simulink library "pixhawk_slib_rfly"  (R2022b)
settings: Solver=ode45  StartTime=0.0  StopTime=10.0  RelTol=1e-3
libraries: pixhawk_slib_uORB_RW x44, $bdroot x7
(part 1 of 2)
settings Model: Creator=skuznick  LastModifiedBy=uavcs
settings SolverCC: AlgebraicLoopSolver=TrustRegion
settings DataIOCC: LimitDataPoints=on  SaveFormat=Array  ReturnWorkspaceOutputs=off
settings OptimizationCC: BlockReduction=off  BooleanDataType=off  LifeSpan=inf
settings DebuggingCC: SaveWithParameterizedLinksMsg=none  UnderspecifiedInitializationDetection=Classic  MergeDetectMultiDrivingBlocksExec=none  SignalResolutionControl=TryResolveAllWithWarning  UnconnectedInputMsg=warning  UnconnectedOutputMsg=warning  UnconnectedLineMsg=warning  AllowSymbolicDim=off  SFUnexpectedBacktrackingDiag=warning  SFNoUnconditionalDefaultTransitionDiag=warning  SFExecutionAtInitializationDiag=none  SFMachineParentedDataDiag=warning  ArithmeticOperatorsInVariantConditions=warning
settings HardwareCC: ProdBitPerPointer=32  ProdBitPerSizeT=32  ProdBitPerPtrDiffT=32  ProdLargestAtomicFloat=None  ProdIntDivRoundTo=Undefined  ProdEndianess=Unspecified  ProdWordSize=32  ProdHWDeviceType=32-bit Generic  TargetUnknown=on
settings ModelReferenceCC: EnableRefExpFcnMdlSchedulingChecks=on  PropagateSignalLabelsOutOfModel=off
settings SFSimCC: SimUseLocalCustomCode=off  CustomCodeUndefinedFunction=UseInterfaceOnly
settings RTWCC: RTWUseLocalCustomCode=off
settings CodeAppCC: StateflowObjectComments=on
settings GRTTargetCC: TargetLangStandard=C89/C90 (ANSI)
settings ConfigComp: CovMetricSettings=dw  CovSaveCumulativeToWorkspaceVar=on  CovSaveSingleToWorkspaceVar=on  CovExternalEMLEnable=off  CovSFcnEnable=off

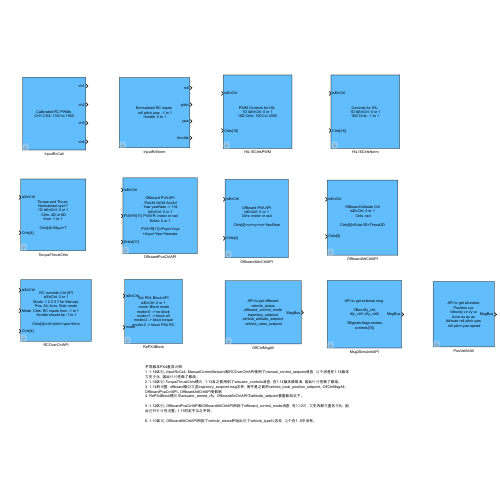
[thumbnail: Simulink's stored preview of the top-level diagram]
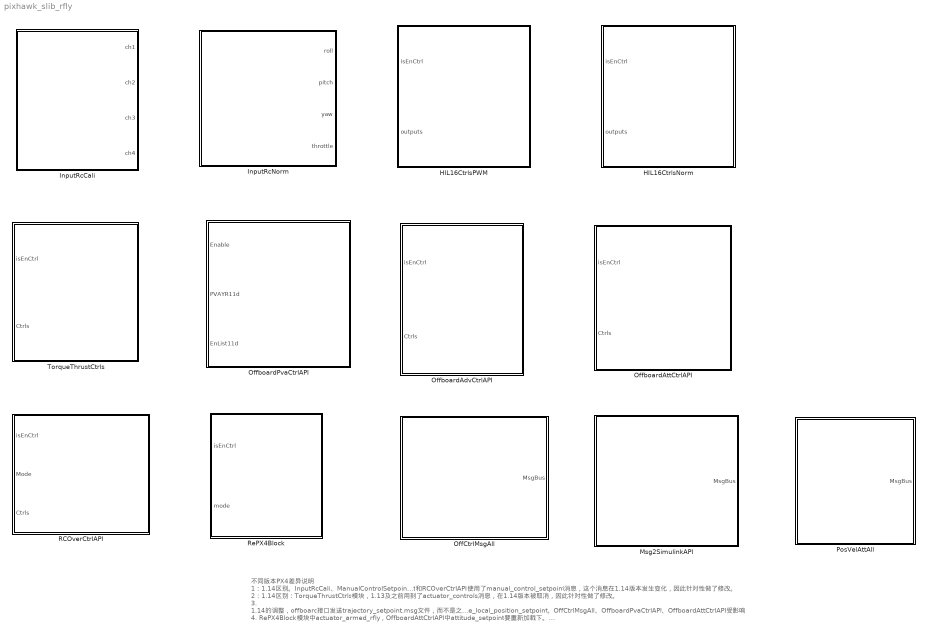
== system pixhawk_slib_rfly ==
  note: 不同版本PX4差异说明
      | 1：1.14区别。InputRcCali、ManualControlSetpoint和RCOverCtrlAPI使用了manual_control_setpoint消息，这个消息在1.14版本发生变化，因此针对性做了修改。
      | 2：1.14区别：TorqueThrustCtrls模块，1.13及之前用到了actuator_controls消息，在1.14版本被取消，因此针对性做了修改。
      | 3. 1.14的调整，offboard接口发送trajectory_setpoint.msg文件，而不是之前的vehicle_local_position_setpoint。OffCtrlMsgAll、OffboardPvaCtrlAPI、OffboardAttCtrlAPI受影响
      | 4. RePX4Block模块中actuator_armed_rfly，OffboardAttCtrlAPI中attitude_setpoint要重新加载下。
      |
      | 5：1.12区别。OffboardPvaCtrlAPI和OffboardAttCtrlAPI用到了offboard_control_mode消息，在1.12时，发生内部变量名变化，因此进行针对性调整。1.11的定于与之不同。
      |
      | 6. 1.10区别，OffboardAttCtrlAPI用到了vehicle_status开始出现了vehicle_type标志位，这个在1.,9中没有。
  HIL16CtrlsNorm : Subsystem  mask{isAutoArm=on, isAutoBlock=on, isAutoLoiter=on, SamTime=-1}
      mask prompts: isAutoArm "Auto arm"; isAutoBlock "Auto block PX4"; isAutoLoiter "Auto Loiter"; SamTime "Sample Time (s)"
      mask help:
      | This block outputs 16D normalized control signals Ctrls[16] for HIL simulation with range from -1 to 1
      |
      | If the input port isEnCtrl is true, the Ctrls will be sent; otherwise zeros output [0,...,0] will be sent.
      |
      | Notice:
      | For multicopter, Ctrls[i] is  usually with range 0 to 1
      | For fixed-wing, Ctrls[i] is  usually with range -1 to 1
      | Note: the throttle channel should also be -1 to 1 for 0% to 100% throttle
      |
      | The output Ctrls will be eventually sent to inPWMs of CopterSim's DLL model.
      |
      | In configuration page:
      | If "Auto arm" is checked, the module will send arm command when isEnCtrl is enabled
      | If "Auto block PX4" is checked, the module will send signals to block PX4's output  when isEnCtrl is enabled, which makes sure this Simulink controller can control the vehicle.
      | If "Auto Loiter" is checked, the module will send cmd to unblock PX4 and switch to auto loiter mode when isEnCtrl is disabled, which makes sure the vehicle can switch to PX4 controller and stay in the air.
      mask init:
      | SamTime=double(SamTime);
      mask Help: eval('sharedhelp(''HIL16CtrlsNorm'')');
      mask Display:
      | fprintf('Controls for HIL \n 1D isEnCtrl: 0 or 1 \n 16D Ctrls: -1 to 1 ')
      | 
      | port_label('input', 1, 'isEnCtrl');
      | port_label('input', 2, 'Ctrls[16]');
  HIL16CtrlsPWM : Subsystem  mask{isAutoArm=on, isAutoBlock=on, isAutoLoiter=on, SamTime=-1}
      mask prompts: isAutoArm "Auto arm"; isAutoBlock "Auto block PX4"; isAutoLoiter "Auto Loiter"; SamTime "Sample Time (s)"
      mask help:
      | This block outputs 16D PWM control signals Ctrls[16] for HIL simulation with range from 1000 to 2000
      |
      | This model has the same function as PWM_output if "Publish Outputs" is checked
      |
      | If the input port isEnCtrl is true, the Ctrls will be sent; otherwise [1000,...,1000] will be sent.
      |
      | In configuration page:
      | If "Auto arm" is checked, the module will send arm command when isEnCtrl is enabled
      | If "Auto block PX4" is checked, the module will send signals to block PX4's output  when isEnCtrl is enabled, which makes sure this Simulink controller can control the vehicle.
      | If "Auto Loiter" is checked, the module will send cmd to unblock PX4 and switch to auto loiter mode when isEnCtrl is disabled, which makes sure the vehicle can switch to PX4 controller and stay in the air.
      |
      | Notice:
      | For multicopter, Ctrls[i]=1000-2000 will be eventually mapped to inPWMs[i] of CopterSim DLL  with range 0 to 1
      | For fixed-wing, Ctrls[i]=1000-2000 will be eventually mapped to inPWMs[i] of CopterSim DLL   with range -1 to 1
      mask init:
      | SamTime=double(SamTime);
      mask Help: eval('sharedhelp(''HIL16CtrlsPWM'')');
      mask Display:
      | fprintf('PWM Controls for HIL \n 1D isEnCtrl: 0 or 1 \n 16D Ctrls: 1000 to 2000 ')
      | 
      | port_label('input', 1, 'isEnCtrl');
      | port_label('input', 2, 'Ctrls[16]');
  InputRcCali : Subsystem  mask{SamTime=1/250.0}
      mask prompts: SamTime "Sample time (s)"
      mask help:
      | This block outputs cablibrated RC pwms for ch1 to ch4 with range 1100 to 1900
      | 1100 1500 and 1900 are the low, central and high stick position
      | CH1 is the roll channel, 1900 for rightwards
      | CH2 is the pitch channel, 1900 for backwards
      | CH3 is the throttle channel, 1900 for upwards
      | CH4 is the yaw channel, 1900 for rightwards spin
      mask init:
      | SamTime=double(SamTime);
      mask Help: eval('sharedhelp(''InputRcCali'')');
      mask Display:
      | fprintf('Calibrated RC PWMs \n CH1-CH4: 1100 to 1900 ')
      | 
      | port_label('output', 1, 'ch1');
      | port_label('output', 2, 'ch2');
      | port_label('output', 3, 'ch3');
      | port_label('output', 4, 'ch4');
  InputRcNorm : Subsystem  mask{ThrType=[0,1]: 0 for 0% throttle and 1 for 100% throttle, SamTime=1/250}
      mask prompts: ThrType "Throttle range type:"; SamTime "Sample Time (s)"
      mask help:
      | This block outputs the normalized control signals from RC
      |
      | roll: [-1,1] move right,   positive roll rotation,  right side down
      |
      | pitch: [-1,1] move forward, negative pitch rotation, nose down
      |
      | yaw: [-1,1] positive yaw rotation,   clockwise when seen top down
      |
      | throttle:  [0,1] for 0% to 100% throttle，move up when throttle>0.5 throttle
      | or  [-1,1] for 0% to 100% throttle，move up when throttle>0 throttle
      mask init:
      | SamTime=double(SamTime);
      mask Help: eval('sharedhelp(''InputRcNorm'')');
      mask TypeOptions ThrType: [0,1]: 0 for 0% throttle and 1 for 100% throttle | [-1,1]: -1 for 0% throttle and 1 for 100% throttle
      mask Display:
      | port_label('output', 1, 'roll');
      | port_label('output', 2, 'pitch');
      | port_label('output', 3, 'yaw');
      | port_label('output', 4, 'throttle');
      | 
      | ThrType = get_param(gcb,'ThrType');
      | if contains(ThrType,'[0,1]')
      |     fprintf('Normalized RC inputs \n roll pitch yaw: -1 to 1\n throttle: 0 to 1')
      | else
      |     fprintf('Normalized RC inputs \n roll pitch yaw: -1 to 1\n throttle: -1 to 1')
      | end
  Msg2SimulinkAPI : Subsystem  mask{SamTime=1/250}
      mask prompts: SamTime "Sample Time (s)"
      mask Help: eval('sharedhelp(''Msg2SimulinkAPI'')');
      mask Display:
      | fprintf('API to get external msg \n\n 3Bus:rfly_ctrl,\n rfly_ctrl1,rfly_ctrl2 \n\n 3Signals:flags,modes,\n controls[16]	')
      | 
      | port_label('output', 1, 'MsgBus');
  OffCtrlMsgAll : Subsystem  mask{SamTime=1/250}
      mask prompts: SamTime "Sample Time (s)"
      mask Help: eval('sharedhelp(''OffCtrlMsgAll'')');
      mask Display:
      | fprintf('API to get offboard\n vehicle_status \n offboard_control_mode \n trajectory_setpoint \n vehicle_attitude_setpoint \n vehicle_rates_setpoint')
      | 
      | port_label('output', 1, 'MsgBus');
  OffboardAdvCtrlAPI : Subsystem  mask{isX=off, isY=off, isZ=off, isVx=on, isVy=on, isVz=on, isAx=off, isAy=off, isAz=off, isYaw=off, isYawRate=on, isOffEnList=zeros(11,1), EnIdxList=[1], isAutoArm=on, isAutoBlock=on, isAutoLoiter=on, SamTime=-1}
      mask prompts: isX "x"; isY "y"; isZ "z"; isVx "vx"; isVy "vy"; isVz "vz"; isAx "ax"; isAy "ay"; isAz "az"; isYaw "yaw"; isYawRate "yawrate"; isOffEnList "isEnList"; EnIdxList "mapList"; isAutoArm "Auto arm and offboard"; isAutoBlock "Auto unblock PX4"; isAutoLoiter "Auto Loiter"; SamTime "Sample Time (s)"
      mask help:
      | You can check the channels and prepare an input signal Ctrls with dimension and sequence corresponding to the of the checked channels.
      |
      | This Block enable offboard control for x y z vx vy vz ax ay az yaw yawrate
      |
      | If the input port isEnCtrl is true, the Ctrls will be sent; otherwise Ctrls will not be sent and PX4 will change to Loiter mode
      |
      | # Needs to be kinematically consistent and feasible for smooth flight.
      | # setting a value to NaN means the state should not be controlled
      |
      | # NED local world frame
      | x,y,z: position # in meters
      | Vx,Vy,Vz: velocity # in meters/second
      | Ax,Ay,Az: acceleration # in meters/second^2
      | yaw: euler angle of desired attitude in radians -PI..+PI
      | yawspeed: angular velocity around NED frame z-axis in radians/second
      |
      | In configuration page:
      | If "Auto arm and offboard" is checked, the module will send arm command and switch to offboard mode (with a 1.5s delay) when isEnCtrl is enabled
      | If "Auto unblock PX4" is checked, the module will send signals to unblock PX4's controls, which makes sure this Simulink controller can control the vehicle throught PX4's Offboard API.
      | If "Auto Loiter" is checked, the module will send cmd to switch to auto loiter mode when isEnCtrl is disabled, which makes sure the vehicle can switch to PX4 controller and stay in the air.
      mask init:
      | isOffEnList=boolean([isX,isY,isZ,isVx,isVy,isVz,isAx,isAy,isAz,isYaw,isYawRate]);
      | 
      | EnIdxList=[];
      | for i=1:length(isOffEnList)
      |     if isOffEnList(i)
      |         EnIdxList=[EnIdxList,i];
      |     end
      | end
      | 
      | SamTime=double(SamTime);
      mask Help: eval('sharedhelp(''OffboardAdvCtrlAPI'')');
      mask DialogControl Control2 Prompt: Select channels to control
      mask DialogControl Container3 Prompt: Option Functions
      mask Display:
      | nameList=["x";"y";"z";"vx";"vy";"vz";"ax";"ay";"az";"Yaw";"YawRate"];
      | nameList2=["isX";"isY";"isZ";"isVx";"isVy";"isVz";"isAx";"isAy";"isAz";"isYaw";"isYawRate"];
      | 
      | idx=0;
      | DispName='';
      | for i=1:length(nameList2)
      |     str0=char(nameList2(i));
      |     if strcmp(get_param(gcb,str0),'on') == true
      |         idx=idx+1;
      |         if idx==1
      |             DispName=[DispName,'',char(nameList(i))];
      |         else
      |             DispName=[DispName,'+',char(nameList(i))];
      |         end
      | 
      |         if mod(idx,4)==0
      |             DispName=[DispName,'\n'];
      |         end
      |     end
      | end
      | 
      | 
      | port_label('input', 1, 'isEnCtrl');
      | port_label('input', 2, ['Ctrls[',num2str(idx),']']);
      | 
      | fprintf(['Offboard PVA API\n isEnCtrl: 0 or 1 \n Ctrls: meter or rad \n\n','Ctrls[',num2str(idx),']=',DispName]);
      | 
      | set_param([gcb,'/Ctrls'],'PortDimensions',num2str(idx));
      | %set_param([gcb,'/OffboardAdvCtrlAPI'],'PortDimensions',num2str(idx));
  OffboardAttCtrlAPI : Subsystem  mask{isAtti=on, EulerOrQuat=Euler3D: roll pitch yaw (rad), isEuler=on, isQuat=off, isRollR=off, isPitchR=off, isYawR=off, isThrust=on, isEnList=[0 0 0 0 0 0], isMapList=[1,2,3], isAutoArm=on, isAutoBlock=on, isAutoLoiter=on, SamTime=-1}
      mask prompts: isAtti "Attitude"; isEuler "Attitude Euler 3D (rad)"; isQuat "Attitude Quaternion 4D"; isRollR "RollRate 1D (rad/s)"; isPitchR "PitchRate 1D (rad/s)"; isYawR "YawRate 1D (rad/s)"; isThrust "Thrust3D Norm"; isEnList "Enlist"; isMapList "MapList"; isAutoArm "Auto arm and offboard"; isAutoBlock "Auto unblock PX4"; isAutoLoiter "Auto Loiter"; SamTime "Sample Time (s)"
      mask help:
      | You can check the channels and prepare an input signal Ctrls with dimension and sequence corresponding to the of the checked channels.
      |
      | isEnCtrl is true, the Ctrls will be sent; otherwise Ctrls will not be sent and PX4 will change to Loiter mode
      | Euler3D=[roll_body, pitch_body, yaw_body] in rad
      | Quat4D: desired quaternion for quaternion control
      | thrust3D: Normalized thrust command in body NED frame [-1,1]
      | # For clarification: For multicopters thrust[0] and thrust[1] are usually 0 and thrust[2] is the negative throttle demand.
      | # For fixed wings thrust[0] is the throttle demand and thrust[1], thrust[2] will usually be zero.
      |
      | In configuration page:
      | If "Auto arm and offboard" is checked, the module will send arm command and switch to offboard mode (with a 1.5s delay) when isEnCtrl is enabled
      | If "Auto unblock PX4" is checked, the module will send signals to unblock PX4's controls, which makes sure this Simulink controller can control the vehicle throught PX4's Offboard API.
      | If "Auto Loiter" is checked, the module will send cmd to switch to auto loiter mode when isEnCtrl is disabled, which makes sure the vehicle can switch to PX4 controller and stay in the air.
      mask init:
      | isEnList=boolean([isEuler isQuat isRollR isPitchR isYawR,isThrust]);
      | isMapList=[];
      | 
      | if isEuler>0.5
      |     isMapList=[isMapList,1,2,3];
      | elseif isQuat>0.5
      |     isMapList=[isMapList,4,5,6,7];
      | end
      | 
      | if isRollR>0.5
      |     isMapList=[isMapList,8];
      | end
      | 
      | if isPitchR>0.5
      |     isMapList=[isMapList,9];
      | end
      | 
      | if isYawR>0.5
      |     isMapList=[isMapList,10];
      | end
      | 
      | if isThrust>0.5
      |     isMapList=[isMapList,11,12,13];
      | end
      | 
      | 
      | SamTime=double(SamTime);
      mask Help: eval('sharedhelp(''OffboardAttCtrlAPI'')');
      mask Callback isAtti:
      | maskObj = Simulink.Mask.get(gcb);
      | for i=1:length(maskObj.Parameters)
      |     if strcmp(maskObj.Parameters(i).Name,'EulerOrQuat')
      |         if strcmp(get_param(gcb,'isAtti'),'on')
      |             maskObj.Parameters(i).Enabled='on';
      |         else
      |             maskObj.Parameters(i).Enabled='off';
      |         end
      |     end
      | end
      | 
      | 
      | set_param(gcb,'isEuler','off');
      | set_param(gcb,'isQuat','off');
      | if strcmp(get_param(gcb,'isAtti'),'on')
      | if contains(get_param(gcb,'EulerOrQuat'),'Euler3D')
      |         set_param(gcb,'isEuler','on');
      |     else
      |         set_param(gcb,'isQuat','on');
      |     end
      | end
      mask TypeOptions EulerOrQuat: Euler3D: roll pitch yaw (rad) | Quat4D: w x y z
      mask Callback EulerOrQuat:
      | set_param(gcb,'isEuler','off');
      | set_param(gcb,'isQuat','off');
      | if strcmp(get_param(gcb,'isAtti'),'on')
      |     if contains(get_param(gcb,'EulerOrQuat'),'Euler3D')
      |         set_param(gcb,'isEuler','on');
      |     else
      |         set_param(gcb,'isQuat','on');
      |     end
      | end
      mask DialogControl Control2 Prompt: This Block enable offboard attitude control api for angle, rate and thrust control
      mask DialogControl Container3 Prompt: Option Functions
      mask Display:
      | nameList=["Euler3D";"Quat4D";"RollRate1D";"PitchRate1D";"YawRate1D";"Thrust3D"];
      | nameList2=["isEuler";"isQuat";"isRollR";"isPitchR";"isYawR";"isThrust"];
      | lenList=[3,4,1,1,1,3];
      | 
      | idx=0;
      | idx2=0;
      | DispName='';
      | for i=1:length(nameList2)
      |     str0=char(nameList2(i));
      |     if strcmp(get_param(gcb,str0),'on') == true
      |         idx=idx+lenList(i);
      |         idx2=idx2+1;
      |         if idx2==1
      |             DispName=[DispName,'',char(nameList(i))];
      |         else
      |             DispName=[DispName,'+',char(nameList(i))];
      |         end
      | 
      |         if mod(idx2,2)==0
      |             DispName=[DispName,'\n'];
      |         end
      |     end
      | end
      | 
      | 
      | port_label('input', 1, 'isEnCtrl');
      | port_label('input', 2, ['Ctrls[',num2str(idx),']']);
      | 
      | set_param([gcb,'/Ctrls'],'PortDimensions',num2str(idx));
      | 
      | fprintf(['Offboard Attitude Ctrl\n isEnCtrl: 0 or 1 \n Ctrls: rad\n\n','Ctrls[',num2str(idx),']=',DispName]);
  OffboardPvaCtrlAPI : Subsystem  mask{isAutoArm=on, isAutoBlock=on, isAutoLoiter=on, SamTime=-1}
      mask prompts: isAutoArm "Auto arm and offboard"; isAutoBlock "Auto unblock PX4"; isAutoLoiter "Auto Loiter"; SamTime "Sample Time (s)"
      mask help:
      | This Block enable offboard control for x y z vx vy vz ax ay az yaw yawrate
      |
      | If the input port isEnCtrl is true, the Ctrls will be sent; otherwise Ctrls will not be sent and PX4 will change to Loiter mode
      |
      | # Needs to be kinematically consistent and feasible for smooth flight.
      | # setting a value to NaN means the state should not be controlled
      |
      | # NED local world frame
      | x,y,z: position # in meters
      | Vx,Vy,Vz: velocity # in meters/second
      | Ax,Ay,Az: acceleration # in meters/second^2
      | yaw: euler angle of desired attitude in radians -PI..+PI
      | yawspeed: angular velocity around NED frame z-axis in radians/second
      |
      | In configuration page:
      | If "Auto arm and offboard" is checked, the module will send arm command and switch to offboard mode (with a 1.5s delay) when isEnCtrl is enabled
      | If "Auto unblock PX4" is checked, the module will send signals to unblock PX4's controls, which makes sure this Simulink controller can control the vehicle throught PX4's Offboard API.
      | If "Auto Loiter" is checked, the module will send cmd to switch to auto loiter mode when isEnCtrl is disabled, which makes sure the vehicle can switch to PX4 controller and stay in the air.
      mask init:
      | SamTime=double(SamTime);
      mask Help: eval('sharedhelp(''OffboardPvaCtrlAPI'')');
      mask Display:
      | fprintf('Offboard PVA API\n Pos3d Vel3d Acc3d\n Yaw yawRate -> 11d\n isEnCtrl: 0 or 1 \n PVAYR: meter or rad\n Enlist: 0 or 1 \n\n PVAYR[11]=Pxyz+Vxyz\n+Axyz+Yaw+Yawrate')
      | 
      | port_label('input', 1, 'isEnCtrl');
      | port_label('input', 2, 'PVAYR[11]');
      | port_label('input', 3, 'Enlist[11]');
  PosVelAttAll : Subsystem  mask{SamTime=1/250}
      mask prompts: SamTime "Sample Time (s)"
      mask Help: eval('sharedhelp(''PosVelAttAll'')');
      mask Display:
      | fprintf('API to get all states\n Position xyz \n Velocity vx vy vz \n Acce ax ay ax \n Attitude roll pitch yaw \n roll pitch yaw speed')
      | 
      | port_label('output', 1, 'MsgBus');
  RCOverCtrlAPI : Subsystem  mask{isRoll=on, isPitch=on, isYaw=on, isThrottle=on, isFlaps=off, isAux1=off, isAux2=off, isAux3=off, isAux4=off, isAux5=off, isAux6=off, isOffEnList=[0 0 0 0 0 0], EnIdxList=[1,2,3], isAutoArm=on, isAutoBlock=on, isAutoLoiter=on, SamTime=-1}
      mask prompts: isRoll "roll"; isPitch "pitch"; isYaw "yaw"; isThrottle "throttle"; isFlaps "flaps"; isAux1 "aux1"; isAux2 "aux2"; isAux3 "aux3"; isAux4 "aux4"; isAux5 "aux5"; isAux6 "aux6"; isOffEnList "Enlist"; EnIdxList "MapList"; isAutoArm "Auto arm"; isAutoBlock "Auto unblock PX4"; isAutoLoiter "Auto Loiter"; SamTime "Sample Time (s)"
      mask help:
      | This block relealizes the manual_control_setpoint to prvovide an API to generate RC control signals by Simulink controller.
      |
      | Mode=1: MANUAL, Mode=2: ALTCTL,        Mode=3: POSCTL
      | Mode=5: ACRO,   Mode=7: STABILIZED
      |
      | Ctrls
      | roll: [-1,1] move right,   positive roll rotation,  right side down
      | pitch: [-1,1] move forward, negative pitch rotation, nose down
      | yaw: [-1,1] positive yaw rotation,   clockwise when seen top down
      | throttle:  [-1,1] for 0% to 100% throttle，move up when positive throttle
      |
      | In configuration page:
      | If "Auto arm and offboard" is checked, the module will send arm command and switch to offboard mode (with a 1.5s delay) when isEnCtrl is enabled
      | If "Auto unblock PX4" is checked, the module will send signals to unblock PX4's controls, which makes sure this Simulink controller can control the vehicle throught PX4's RC API.
      | If "Auto Loiter" is checked, the module will send cmd to switch to auto loiter mode when isEnCtrl is disabled, which makes sure the vehicle can switch to PX4 controller and stay in the air.
      mask init:
      | SamTime=double(SamTime);
      | 
      | isOffEnList=[isRoll,isPitch,isYaw,isThrottle,isFlaps,isAux1,isAux2,isAux3,isAux4,isAux5,isAux6];
      | 
      | EnIdxList=[];
      | for i=1:length(isOffEnList)
      |     if isOffEnList(i)>0.5
      |         EnIdxList=[EnIdxList,i];
      |     end
      | end
      mask Help: eval('sharedhelp(''RCOverCtrlAPI'')');
      mask DialogControl Control2 Prompt: This Block enable offboard attitude control api for angle, rate and thrust control
      mask Display:
      | %fprintf('RC override Ctrl API\n isEnCtrl: 0 or 1 \nMode: 1 2 3 5 7 for Manual,\nPos, Alt, Acro, Stab mode\n Ctrls: RC inputs from -1 to 1')
      | 
      | nameList=["roll";"pitch";"yaw";"throt";"flaps";"aux1";"aux2";"aux3";"aux4";"aux5";"aux6"];
      | nameList2=["isRoll","isPitch","isYaw","isThrottle","isFlaps","isAux1","isAux2","isAux3","isAux4","isAux5","isAux6"];
      | 
      | idx=0;
      | DispName='';
      | for i=1:length(nameList2)
      |     str0=char(nameList2(i));
      |     if strcmp(get_param(gcb,str0),'on') == true
      |         idx=idx+1;
      |         if idx==1
      |             DispName=[DispName,'',char(nameList(i))];
      |         else
      |             DispName=[DispName,'+',char(nameList(i))];
      |         end
      | 
      |         if mod(idx,4)==0
      |             DispName=[DispName,'\n'];
      |         end
      |     end
      | end
      | 
      | 
      | port_label('input', 1, 'isEnCtrl');
      | port_label('input', 2, 'Mode');
      | port_label('input', 3, ['Ctrls[',num2str(idx),']']);
      | 
      | fprintf(['RC override Ctrl API\n isEnCtrl: 0 or 1 \nMode: 1 2 3 5 7 for Manual,\nPos, Alt, Acro, Stab mode\n Ctrls: RC inputs from -1 to 1 \n throttle should be -1 to 1\n\n','Ctrls[',num2str(idx),']=',DispName]);
      | 
      | set_param([gcb,'/Ctrls'],'PortDimensions',num2str(idx));
  RePX4Block : Subsystem  mask{SamTime=-1}
      mask prompts: SamTime "Sample Time (s)"
      mask help:
      | This API can reset the PX4 blocking option for switching between PX4 offical controller and Simulink controller
      |
      | mode = 0: use PX4 controller and block simulink controller
      |
      | mode =1: block PX4 controller and use simulink controller
      |
      | mode =2: only block actuator_controls_0 (torque and thrust controller) of PX4, you should use "TorqueThrustCtrls" module to send requied control signals
      |
      | mode =3: Block RC's mannul_control_setpoint publish code, this is for RCOverCtrlAPI module.
      mask init:
      | SamTime=double(SamTime);
      mask Help: eval('sharedhelp(''RePX4Block'')');
      mask Display:
      | fprintf('Set PX4 Block API\n isEnCtrl: 0 or 1 \n mode: Block mode\nmode=0 -> no block\nmode=1 -> block all\nmode=2 -> block torque\nmode=2 -> block PX4 RC')
      | 
      | port_label('input', 1, 'isEnCtrl');
      | port_label('input', 2, 'mode');
  TorqueThrustCtrls : Subsystem  mask{is3DThrust=1D Thrust throttle T  (T >0 fly upward);  Input: 4D Ctrls[4], isEnSecond=off, isAutoArm=on, isAutoBlock=on, isAutoLoiter=on, SamTime=-1, ctrlIdxList=0, SignList=0}
      mask prompts: is3DThrust "3D Torque Mxyz + 1D Throttle or 3D Force"; isEnSecond "Enable 2nd channel (for VOTLs): Ctrls should be 8D or 12D"; isAutoArm "Auto arm"; isAutoBlock "Auto block PX4"; isAutoLoiter "Auto Loiter"; SamTime "Sample Time (s)"; ctrlIdxList "EnList"
      mask help:
      | This block sends the nominied xyz torque and thrust (1D T or 3D Txxyz)  control signals with range -1 to 1, which will be sent to PX4 mixer to control the motors. For multicopter, there is T=-Txyz(3) and T is [0,1], because Txyz is defined in body FRD frame.
      |
      | If the input port isEnCtrl is true, the Ctrls will be sent; otherwise zeros output [0,...,0] will be sent.
      |
      | Txyz: thrust setpoint along X, Y, Z body axis [-1, 1]  (normalized)
      | Mxyz: torque setpoint about X, Y, Z body axis [-1, 1] (normalized)
      |
      | For PX4 1.7 - 1.13, the Ctrls will send uORB message: actuator_controls_0 and actuator_controls_1 (2nd channel, for VTOL etc)
      |
      | For PX4 1.14 and above,  the Ctrls will send uORB message:  vehicle_torque_setpoint and vehicle_torque_setpoint, and  vehicle_torque_setpoint1 and vehicle_torque_setpoint1 (2nd channel, for VTOL etc)
      |
      | In configuration page:
      | If "Auto arm" is checked, the module will send arm command when isEnCtrl is enabled
      | If "Auto block PX4" is checked, the module will send signals to block PX4's torque and thrust (actuator_controls_0) message  when isEnCtrl is enabled, which makes sure this Simulink controller can control the vehicle.
      | If "Auto Loiter" is checked, the module will send cmd to unblock PX4 and switch to auto loiter mode when isEnCtrl is disabled, which makes sure the vehicle can switch to PX4 controller and stay in the air.
      mask init:
      | SamTime=double(SamTime);
      | 
      | is3DThrust=double(is3DThrust);
      | isEnSecond=double(isEnSecond);
      | 
      | if is3DThrust<1.5
      |     if isEnSecond<0.5
      |         ctrlIdxList=[1 2 3 6];
      |         SignList=[1 1 1 -1];
      |     else
      |         ctrlIdxList=[1 2 3 6 7 8 9 12];
      |         SignList=[1 1 1 -1 1 1 1 -1];
      |     end
      |     
      |     
      | else
      |     if isEnSecond<0.5
      |         ctrlIdxList=[1 2 3 4 5 6];
      |         SignList=[1 1 1 1 1 1];
      |     else
      |         ctrlIdxList=[1 2 3 4 5 6 7 8 9 10 11 12];
      |         SignList=[1 1 1 1 1 1 1 1 1 1 1 1];
      |     end
      | end
      mask Help: eval('sharedhelp(''TorqueThrustCtrls'')');
      mask TypeOptions is3DThrust: 1D Thrust throttle T  (T >0 fly upward);  Input: 4D Ctrls[4] | 3D Thrust force Txyz (Txyz(3)<0 fly upward); Input: 6D Ctrls[6]
      mask DialogControl Container3 Prompt: Option Functions
      mask Display:
      | is3DThrust = get_param(gcb,'is3DThrust');
      | isEnSecond = get_param(gcb,'isEnSecond');
      | 
      | Title='Ctrls[] = Mxyz + Tz';
      | basicCtrl=4;
      | 
      | startStr='Mxyz';
      | if contains(is3DThrust,'Txyz(3)')
      |     basicCtrl=6;
      |     startStr=[startStr,'+Txyz'];
      | else
      |     startStr=[startStr,'+T'];
      | end
      | if strcmp(isEnSecond,'on') == true
      |     basicCtrl=basicCtrl*2;
      |     if contains(is3DThrust,'Txyz(3)')
      |         startStr=[startStr,'+M1xyz+T1xyz'];
      |     else
      |         startStr=[startStr,'+Mxyz+T1'];
      |     end
      | 
      | end
      | 
      | port_label('input', 1, 'isEnCtrl');
      | port_label('input', 2, ['Ctrls[',num2str(basicCtrl),']']);
      | 
      | fprintf(['Torque and Thrust \n Normalized xyz+T \n 1D isEnCtrl: 0 or 1 \n Ctrls: 4D or 6D\n from -1 to 1 \n\n','Ctrls[',num2str(basicCtrl),']=',startStr]);
      | 
      | set_param([gcb,'/Ctrls'],'PortDimensions',num2str(basicCtrl));

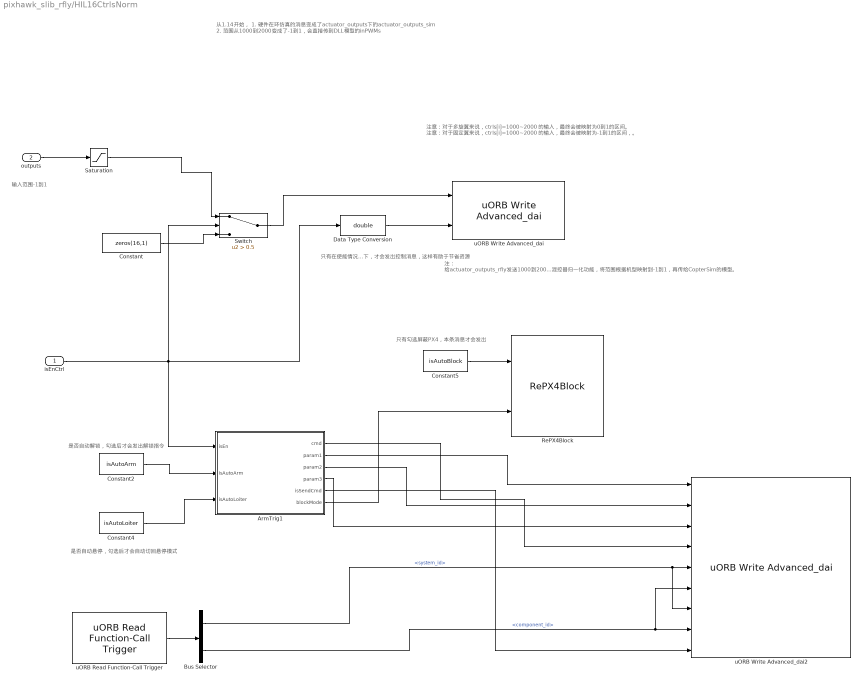
== system pixhawk_slib_rfly/HIL16CtrlsNorm ==
  note: 从1.14开始，
      | 1. 硬件在环仿真的消息变成了actuator_outputs下的actuator_outputs_sim
      | 2. 范围从1000到2000变成了-1到1，会直接传到DLL模型的inPWMs
  note: 输入范围-1到1
  note: 只有在使能情况下，才会发出控制消息，这样有助于节省资源
  note: 是否自动悬停，勾选后才会自动切回悬停模式
  note: 只有勾选屏蔽PX4，本条消息才会发出
  note: 注：
      | 给actuator_outputs_rfly发送1000到2000的数，会在PX4底层（RflySim平台有源码修改）自动触发混控器归一化功能，将范围根据机型映射到-1到1，再传给CopterSim的模型。
  note: 是否自动解锁，勾选后才会发出解锁指令
  note: 注意：对于多旋翼来说，ctrls[i]=1000~2000的输入，最终会被映射为0到1的区间。
      | 注意：对于固定翼来说，ctrls[i]=1000~2000的输入，最终会被映射为-1到1的区间，。
  isEnCtrl : Inport  OutDataTypeStr=boolean  PortDimensions=1
  outputs : Inport  Port=2  OutDataTypeStr=single  PortDimensions=16
  ArmTrig1 : MATLAB Function  TreatAsAtomicUnit=on  SystemSampleTime=SamTime
  Bus Selector : BusSelector  OutputSignals=system_id,component_id
  Constant : Constant  Value=zeros(16,1)  OutDataTypeStr=single
  Constant2 : Constant  Value=isAutoArm  OutDataTypeStr=boolean
  Constant4 : Constant  Value=isAutoLoiter  OutDataTypeStr=boolean
  Constant5 : Constant  Value=isAutoBlock  OutDataTypeStr=boolean
  Data Type Conversion : DataTypeConversion  OutDataTypeStr=double  SaturateOnIntegerOverflow=off  RndMeth=Floor
  RePX4Block : $bdroot/RePX4Block  SamTime=SamTime
  Saturation : Saturate  UpperLimit=1  LowerLimit=-1
  Switch : Switch  Criteria=u2 > Threshold  Threshold=0.5  SaturateOnIntegerOverflow=off  InputSameDT=off
  uORB Read Function-Call Trigger : pixhawk_slib_uORB_RW/uORB Read Function-Call Trigger  uORB_Topic_str='vehicle_status'  BusObjVar=Bus: vehicle_status_SL  uORB_Interval=4  AsyncOutput=off  Fcn_call_select=Generate Function Call Signal  TaskName='Task1'  Poll_timeout=-1  Ts=SamTime
      settings: SourceProductName=Pixhawk Target Blocks
  uORB Write Advanced_dai : pixhawk_slib_uORB_RW/uORB Write Advanced_dai  Ts=0  uORB_AdvtQueue=on  uORB_FieldEnabledArr="0  0  0  1  0  0  0  0  0  0  0"  uORB_Topic_str=0  uORB_Topic_str_ID=0  uORB_Struct_DT="[1  1  1  1  1]"  BlockInputCount=5  uORB_StructParams="[\"voltage_v\",\"voltage_filtered_v\",\"current_a\",\"current_filtered_a\",\"remaining\"]"  uORB_PortSizes="[1  1  1  1]"  MsgSizeOf=0  MW_update=true
      settings: SourceProductName=Pixhawk Target Blocks
  uORB Write Advanced_dai2 : pixhawk_slib_uORB_RW/uORB Write Advanced_dai  Ts=0  uORB_AdvtQueue=on  uORB_FieldEnabledArr="0  0  0  1  0  0  0  0  0  0  0"  uORB_Topic_str=0  uORB_Topic_str_ID=0  uORB_Struct_DT="[1  1  1  1  1]"  BlockInputCount=5  uORB_StructParams="[\"voltage_v\",\"voltage_filtered_v\",\"current_a\",\"current_filtered_a\",\"remaining\"]"  uORB_PortSizes="[1  1  1  1]"  MsgSizeOf=0  MW_update=true
      settings: SourceProductName=Pixhawk Target Blocks
  wires:
  Constant/1 -> Switch/3
  outputs/1 -> Saturation/1
  Saturation/1 -> Switch/1
  Constant4/1 -> ArmTrig1/3(isAutoLoiter)
  uORB Read Function-Call Trigger/1 -> Bus Selector/1
  isEnCtrl/1 -> Switch/2, Data Type Conversion/1, ArmTrig1/1(isEn)
  Constant5/1 -> RePX4Block/1
  ArmTrig1/6(blockMode) -> RePX4Block/2
  Data Type Conversion/1 -> uORB Write Advanced_dai/2
  ArmTrig1/5(isSendCmd) -> uORB Write Advanced_dai2/9
  ArmTrig1/3(param2) -> uORB Write Advanced_dai2/2
  Bus Selector/1 -> uORB Write Advanced_dai2/7, uORB Write Advanced_dai2/5  "<system_id>"
  Bus Selector/2 -> uORB Write Advanced_dai2/8, uORB Write Advanced_dai2/6  "<component_id>"
  ArmTrig1/4(param3) -> uORB Write Advanced_dai2/3
  ArmTrig1/1(cmd) -> uORB Write Advanced_dai2/4
  ArmTrig1/2(param1) -> uORB Write Advanced_dai2/1
  Constant2/1 -> ArmTrig1/2(isAutoArm)
  Switch/1 -> uORB Write Advanced_dai/1

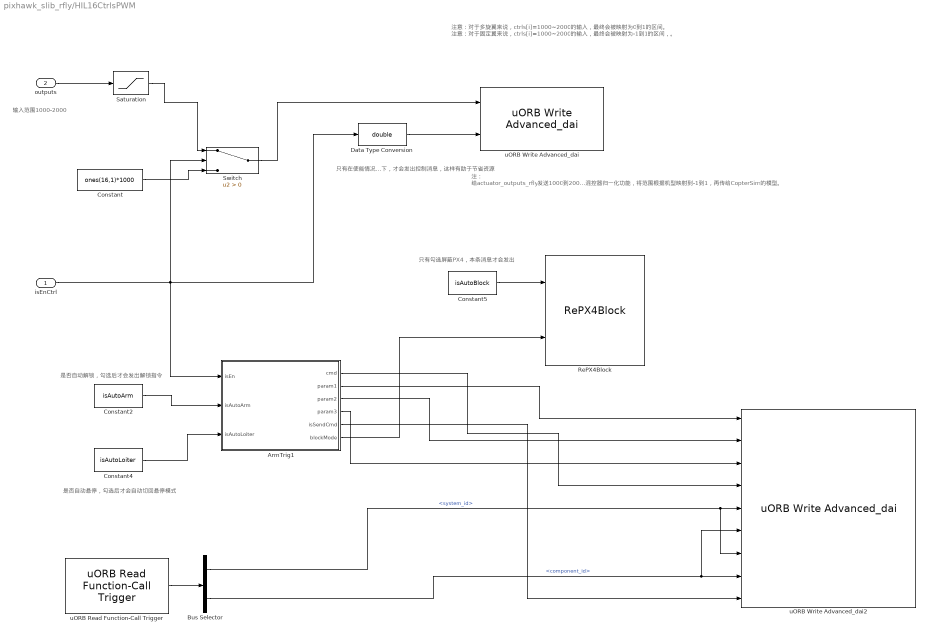
== system pixhawk_slib_rfly/HIL16CtrlsPWM ==
  note: 只有在使能情况下，才会发出控制消息，这样有助于节省资源
  note: 是否自动悬停，勾选后才会自动切回悬停模式
  note: 是否自动解锁，勾选后才会发出解锁指令
  note: 只有勾选屏蔽PX4，本条消息才会发出
  note: 注意：对于多旋翼来说，ctrls[i]=1000~2000的输入，最终会被映射为0到1的区间。
      | 注意：对于固定翼来说，ctrls[i]=1000~2000的输入，最终会被映射为-1到1的区间，。
  note: 注：
      | 给actuator_outputs_rfly发送1000到2000的数，会在PX4底层（RflySim平台有源码修改）自动触发混控器归一化功能，将范围根据机型映射到-1到1，再传给CopterSim的模型。
  note: 输入范围1000-2000
  isEnCtrl : Inport  OutDataTypeStr=boolean  PortDimensions=1
  outputs : Inport  Port=2  OutDataTypeStr=single  PortDimensions=16
  ArmTrig1 : MATLAB Function  TreatAsAtomicUnit=on  SystemSampleTime=SamTime
  Bus Selector : BusSelector  OutputSignals=system_id,component_id
  Constant : Constant  Value=ones(16,1)*1000  OutDataTypeStr=single
  Constant2 : Constant  Value=isAutoArm  OutDataTypeStr=boolean
  Constant4 : Constant  Value=isAutoLoiter  OutDataTypeStr=boolean
  Constant5 : Constant  Value=isAutoBlock  OutDataTypeStr=boolean
  Data Type Conversion : DataTypeConversion  OutDataTypeStr=double  SaturateOnIntegerOverflow=off  RndMeth=Floor
  RePX4Block : $bdroot/RePX4Block  SamTime=SamTime
  Saturation : Saturate  UpperLimit=2000  LowerLimit=1000
  Switch : Switch  Criteria=u2 > Threshold  SaturateOnIntegerOverflow=off  InputSameDT=off
  uORB Read Function-Call Trigger : pixhawk_slib_uORB_RW/uORB Read Function-Call Trigger  uORB_Topic_str='vehicle_status'  BusObjVar=Bus: vehicle_status_SL  uORB_Interval=4  AsyncOutput=off  Fcn_call_select=Generate Function Call Signal  TaskName='Task1'  Poll_timeout=-1  Ts=SamTime
      settings: SourceProductName=Pixhawk Target Blocks
  uORB Write Advanced_dai : pixhawk_slib_uORB_RW/uORB Write Advanced_dai  Ts=0  uORB_AdvtQueue=on  uORB_FieldEnabledArr="0  0  0  1  0  0  0  0  0  0  0"  uORB_Topic_str=0  uORB_Topic_str_ID=0  uORB_Struct_DT="[1  1  1  1  1]"  BlockInputCount=5  uORB_StructParams="[\"voltage_v\",\"voltage_filtered_v\",\"current_a\",\"current_filtered_a\",\"remaining\"]"  uORB_PortSizes="[1  1  1  1]"  MsgSizeOf=0  MW_update=true
      settings: SourceProductName=Pixhawk Target Blocks
  uORB Write Advanced_dai2 : pixhawk_slib_uORB_RW/uORB Write Advanced_dai  Ts=0  uORB_AdvtQueue=on  uORB_FieldEnabledArr="0  0  0  1  0  0  0  0  0  0  0"  uORB_Topic_str=0  uORB_Topic_str_ID=0  uORB_Struct_DT="[1  1  1  1  1]"  BlockInputCount=5  uORB_StructParams="[\"voltage_v\",\"voltage_filtered_v\",\"current_a\",\"current_filtered_a\",\"remaining\"]"  uORB_PortSizes="[1  1  1  1]"  MsgSizeOf=0  MW_update=true
      settings: SourceProductName=Pixhawk Target Blocks
  wires:
  Switch/1 -> uORB Write Advanced_dai/1
  Constant/1 -> Switch/3
  outputs/1 -> Saturation/1
  Saturation/1 -> Switch/1
  uORB Read Function-Call Trigger/1 -> Bus Selector/1
  Bus Selector/2 -> uORB Write Advanced_dai2/8, uORB Write Advanced_dai2/6  "<component_id>"
  Bus Selector/1 -> uORB Write Advanced_dai2/7, uORB Write Advanced_dai2/5  "<system_id>"
  Constant2/1 -> ArmTrig1/2(isAutoArm)
  Constant4/1 -> ArmTrig1/3(isAutoLoiter)
  ArmTrig1/1(cmd) -> uORB Write Advanced_dai2/4
  ArmTrig1/2(param1) -> uORB Write Advanced_dai2/1
  ArmTrig1/3(param2) -> uORB Write Advanced_dai2/2
  ArmTrig1/4(param3) -> uORB Write Advanced_dai2/3
  ArmTrig1/5(isSendCmd) -> uORB Write Advanced_dai2/9
  isEnCtrl/1 -> Data Type Conversion/1, ArmTrig1/1(isEn), Switch/2
  Constant5/1 -> RePX4Block/1
  ArmTrig1/6(blockMode) -> RePX4Block/2
  Data Type Conversion/1 -> uORB Write Advanced_dai/2

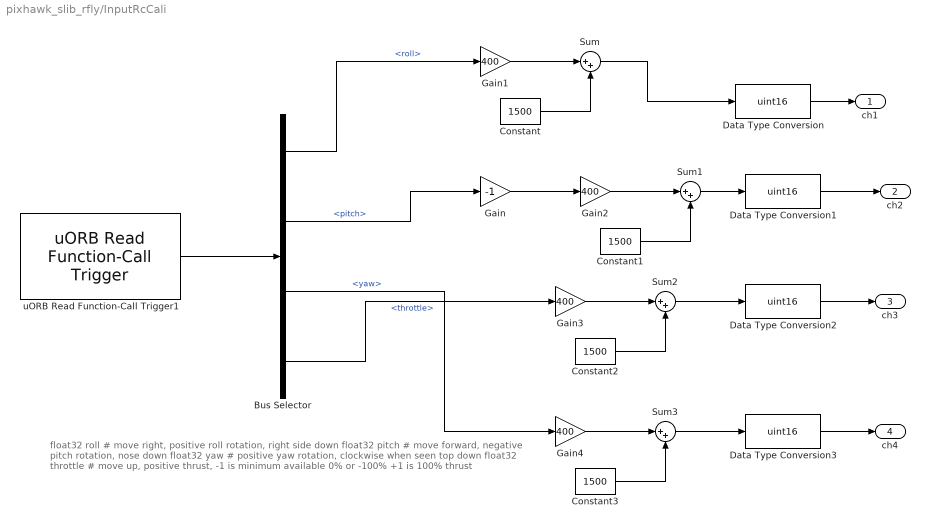
== system pixhawk_slib_rfly/InputRcCali ==
  note: float32 roll     # move right,   positive roll rotation,  right side down
      | float32 pitch    # move forward, negative pitch rotation, nose down
      | float32 yaw      #               positive yaw rotation,   clockwise when seen top down
      | float32 throttle # move up,      positive thrust,         -1 is minimum available 0% or -100% +1 is 100% thrust
  Bus Selector : BusSelector  OutputSignals=roll,pitch,yaw,throttle
  Constant{,1..3} (4 alike) : Constant  Value=1500  OutDataTypeStr=single
  Data Type Conversion{,1..3} (4 alike) : DataTypeConversion  OutDataTypeStr=uint16  SaturateOnIntegerOverflow=off  RndMeth=Floor
  Gain : Gain  Gain=-1
  Gain{1..4} (4 alike) : Gain  Gain=400
  Sum{,1..3} (4 alike) : Sum  Inputs=|++
  uORB Read Function-Call Trigger1 : pixhawk_slib_uORB_RW/uORB Read Function-Call Trigger  uORB_Topic_str='manual_control_setpoint'  BusObjVar=Bus: manual_control_setpoint_SL  uORB_Interval=2  AsyncOutput=off  Fcn_call_select=Generate Function Call Signal  TaskName='Task1'  Poll_timeout=-1  Ts=SamTime
      settings: SourceProductName=Pixhawk Target Blocks
  ch1 : Outport  OutDataTypeStr=uint16  VectorParamsAs1DForOutWhenUnconnected=off
  ch2 : Outport  Port=2  OutDataTypeStr=uint16  VectorParamsAs1DForOutWhenUnconnected=off
  ch3 : Outport  Port=3  OutDataTypeStr=uint16  VectorParamsAs1DForOutWhenUnconnected=off
  ch4 : Outport  Port=4  OutDataTypeStr=uint16  VectorParamsAs1DForOutWhenUnconnected=off
  wires:
  Bus Selector/1 -> Gain1/1  "<roll>"
  Sum/1 -> Data Type Conversion/1
  Sum2/1 -> Data Type Conversion2/1
  Bus Selector/2 -> Gain/1  "<pitch>"
  Sum3/1 -> Data Type Conversion3/1
  Bus Selector/4 -> Gain3/1  "<throttle>"
  Sum1/1 -> Data Type Conversion1/1
  Bus Selector/3 -> Gain4/1  "<yaw>"
  Gain/1 -> Gain2/1
  uORB Read Function-Call Trigger1/1 -> Bus Selector/1
  Gain1/1 -> Sum/1
  Constant/1 -> Sum/2
  Gain2/1 -> Sum1/1
  Constant1/1 -> Sum1/2
  Gain3/1 -> Sum2/1
  Constant2/1 -> Sum2/2
  Gain4/1 -> Sum3/1
  Constant3/1 -> Sum3/2
  Data Type Conversion/1 -> ch1/1
  Data Type Conversion1/1 -> ch2/1
  Data Type Conversion2/1 -> ch3/1
  Data Type Conversion3/1 -> ch4/1

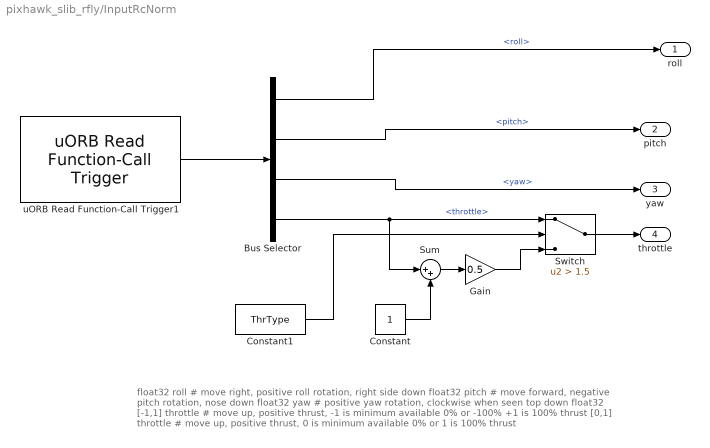
== system pixhawk_slib_rfly/InputRcNorm ==
  note: float32 roll     # move right,   positive roll rotation,  right side down
      | float32 pitch    # move forward, negative pitch rotation, nose down
      | float32 yaw      #               positive yaw rotation,   clockwise when seen top down
      | float32 [-1,1] throttle # move up,      positive thrust,         -1 is minimum available 0% or -100% +1 is 100% thrust
      |  [0,1] throttle # move up,      positive thrust,        0 is minimum available 0% or 1 is 100% thrust
  Bus Selector : BusSelector  OutputSignals=roll,pitch,yaw,throttle
  Constant : Constant  OutDataTypeStr=single
  Constant1 : Constant  Value=ThrType
  Gain : Gain  Gain=0.5
  Sum : Sum  Inputs=|++
  Switch : Switch  Criteria=u2 > Threshold  Threshold=1.5  SaturateOnIntegerOverflow=off  InputSameDT=off
  uORB Read Function-Call Trigger1 : pixhawk_slib_uORB_RW/uORB Read Function-Call Trigger  uORB_Topic_str='manual_control_setpoint'  BusObjVar=Bus: manual_control_setpoint_SL  uORB_Interval=1  AsyncOutput=off  Fcn_call_select=Generate Function Call Signal  TaskName='Task1'  Poll_timeout=-1  Ts=SamTime
      settings: SourceProductName=Pixhawk Target Blocks
  roll : Outport  OutDataTypeStr=single  VectorParamsAs1DForOutWhenUnconnected=off
  pitch : Outport  Port=2  OutDataTypeStr=single  VectorParamsAs1DForOutWhenUnconnected=off
  yaw : Outport  Port=3  OutDataTypeStr=single  VectorParamsAs1DForOutWhenUnconnected=off
  throttle : Outport  Port=4  OutDataTypeStr=single  VectorParamsAs1DForOutWhenUnconnected=off
  wires:
  uORB Read Function-Call Trigger1/1 -> Bus Selector/1
  Gain/1 -> Switch/3
  Bus Selector/1 -> roll/1  "<roll>"
  Bus Selector/2 -> pitch/1  "<pitch>"
  Bus Selector/3 -> yaw/1  "<yaw>"
  Bus Selector/4 -> Sum/1, Switch/1  "<throttle>"
  Constant/1 -> Sum/2
  Sum/1 -> Gain/1
  Constant1/1 -> Switch/2
  Switch/1 -> throttle/1

== system pixhawk_slib_rfly/Msg2SimulinkAPI ==
  Bus Creator : BusCreator  Inputs=3
  rfly_ctrl : pixhawk_slib_uORB_RW/uORB Read Function-Call Trigger  uORB_Topic_str='rfly_ctrl'  BusObjVar=Bus: rfly_ctrl_SL  uORB_Interval=4  AsyncOutput=off  Fcn_call_select=Generate Function Call Signal  TaskName='Task1'  Poll_timeout=-1  Ts=SamTime
      settings: SourceProductName=Pixhawk Target Blocks
  rfly_ctrl1 : pixhawk_slib_uORB_RW/uORB Read Function-Call Trigger  uORB_Topic_str='rfly_ctrl__rfly_ctrl1'  BusObjVar=Bus: rfly_ctrl_SL  uORB_Interval=4  AsyncOutput=off  Fcn_call_select=Generate Function Call Signal  TaskName='Task1'  Poll_timeout=-1  Ts=SamTime
      settings: SourceProductName=Pixhawk Target Blocks
  rfly_ctrl2 : pixhawk_slib_uORB_RW/uORB Read Function-Call Trigger  uORB_Topic_str='rfly_ctrl__rfly_ctrl2'  BusObjVar=Bus: rfly_ctrl_SL  uORB_Interval=4  AsyncOutput=off  Fcn_call_select=Generate Function Call Signal  TaskName='Task1'  Poll_timeout=-1  Ts=SamTime
      settings: SourceProductName=Pixhawk Target Blocks
  MsgBus : Outport  VectorParamsAs1DForOutWhenUnconnected=off
  wires:
  Bus Creator/1 -> MsgBus/1
  rfly_ctrl/1 -> Bus Creator/1  "rfly_ctrl"
  rfly_ctrl1/1 -> Bus Creator/2  "rfly_ctrl1"
  rfly_ctrl2/1 -> Bus Creator/3  "rfly_ctrl2"

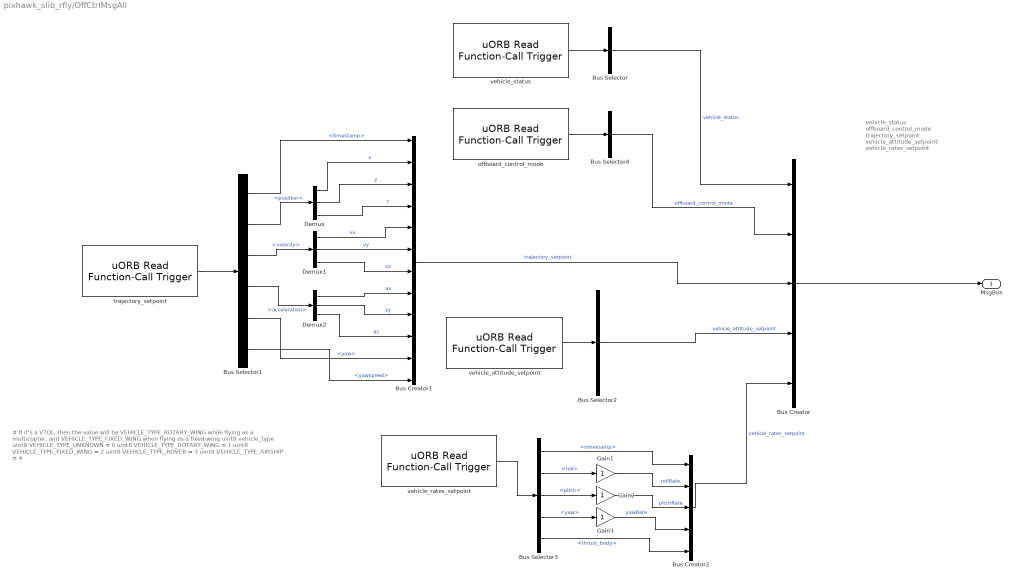
== system pixhawk_slib_rfly/OffCtrlMsgAll ==
  note: vehicle_status
      | offboard_control_mode
      | trajectory_setpoint
      | vehicle_attitude_setpoint
      | vehicle_rates_setpoint
  note: # If it's a VTOL, then the value will be VEHICLE_TYPE_ROTARY_WING while flying as a multicopter, and VEHICLE_TYPE_FIXED_WING when flying as a fixed-wing
      | uint8 vehicle_type
      | uint8 VEHICLE_TYPE_UNKNOWN = 0
      | uint8 VEHICLE_TYPE_ROTARY_WING = 1
      | uint8 VEHICLE_TYPE_FIXED_WING = 2
      | uint8 VEHICLE_TYPE_ROVER = 3
      | uint8 VEHICLE_TYPE_AIRSHIP = 4
  Bus Creator : BusCreator  Inputs=5
  Bus Creator1 : BusCreator  Inputs=12
  Bus Creator2 : BusCreator  Inputs=5
  Bus Selector : BusSelector  OutputSignals=timestamp,arming_state,nav_state,hil_state,vehicle_type,failsafe,is_vtol,system_type,system_id,component_id  OutputAsBus=on
  Bus Selector1 : BusSelector  OutputSignals=timestamp,position,velocity,acceleration,yaw,yawspeed
  Bus Selector2 : BusSelector  OutputSignals=timestamp,roll_body,pitch_body,yaw_body,q_d,thrust_body,yaw_sp_move_rate  OutputAsBus=on
  Bus Selector3 : BusSelector  OutputSignals=timestamp,roll,pitch,yaw,thrust_body
  Bus Selector4 : BusSelector  OutputSignals=timestamp,position,velocity,acceleration,attitude,body_rate  OutputAsBus=on
  Demux : Demux  Outputs=3
  Demux1 : Demux  Outputs=3
  Demux2 : Demux  Outputs=3
  Gain1 : Gain
  Gain2 : Gain
  Gain3 : Gain
  offboard_control_mode : pixhawk_slib_uORB_RW/uORB Read Function-Call Trigger  uORB_Topic_str='offboard_control_mode'  BusObjVar=Bus: offboard_control_mode_SL  uORB_Interval=4  AsyncOutput=off  Fcn_call_select=Generate Function Call Signal  TaskName='Task1'  Poll_timeout=-1  Ts=SamTime
      settings: SourceProductName=Pixhawk Target Blocks
  trajectory_setpoint : pixhawk_slib_uORB_RW/uORB Read Function-Call Trigger  uORB_Topic_str='trajectory_setpoint'  BusObjVar=Bus: trajectory_setpoint_SL  uORB_Interval=4  AsyncOutput=off  Fcn_call_select=Generate Function Call Signal  TaskName='Task1'  Poll_timeout=-1  Ts=SamTime
      settings: SourceProductName=Pixhawk Target Blocks
  vehicle_attitude_setpoint : pixhawk_slib_uORB_RW/uORB Read Function-Call Trigger  uORB_Topic_str='vehicle_attitude_setpoint'  BusObjVar=Bus: vehicle_attitude_setpoint_SL  uORB_Interval=4  AsyncOutput=off  Fcn_call_select=Generate Function Call Signal  TaskName='Task1'  Poll_timeout=-1  Ts=SamTime
      settings: SourceProductName=Pixhawk Target Blocks
  vehicle_rates_setpoint : pixhawk_slib_uORB_RW/uORB Read Function-Call Trigger  uORB_Topic_str='vehicle_rates_setpoint'  BusObjVar=Bus: vehicle_rates_setpoint_SL  uORB_Interval=4  AsyncOutput=off  Fcn_call_select=Generate Function Call Signal  TaskName='Task1'  Poll_timeout=-1  Ts=SamTime
      settings: SourceProductName=Pixhawk Target Blocks
  vehicle_status : pixhawk_slib_uORB_RW/uORB Read Function-Call Trigger  uORB_Topic_str='vehicle_status'  BusObjVar=Bus: vehicle_status_SL  uORB_Interval=4  AsyncOutput=off  Fcn_call_select=Generate Function Call Signal  TaskName='Task1'  Poll_timeout=-1  Ts=SamTime
      settings: SourceProductName=Pixhawk Target Blocks
  MsgBus : Outport  VectorParamsAs1DForOutWhenUnconnected=off
  wires:
  vehicle_rates_setpoint/1 -> Bus Selector3/1
  Bus Creator/1 -> MsgBus/1
  trajectory_setpoint/1 -> Bus Selector1/1
  vehicle_status/1 -> Bus Selector/1
  Bus Creator2/1 -> Bus Creator/5  "vehicle_rates_setpoint"
  Bus Creator1/1 -> Bus Creator/3  "trajectory_setpoint"
  Bus Selector/1 -> Bus Creator/1  "vehicle_status"
  vehicle_attitude_setpoint/1 -> Bus Selector2/1
  Bus Selector4/1 -> Bus Creator/2  "offboard_control_mode"
  offboard_control_mode/1 -> Bus Selector4/1
  Bus Selector1/2 -> Demux/1  "<position>"
  Bus Selector1/3 -> Demux1/1  "<velocity>"
  Bus Selector1/4 -> Demux2/1  "<acceleration>"
  Bus Selector1/1 -> Bus Creator1/1  "<timestamp>"
  Demux/1 -> Bus Creator1/2  "x"
  Demux/2 -> Bus Creator1/3  "y"
  Demux/3 -> Bus Creator1/4  "z"
  Demux1/1 -> Bus Creator1/5  "vx"
  Demux1/2 -> Bus Creator1/6  "vy"
  Demux1/3 -> Bus Creator1/7  "vz"
  Demux2/1 -> Bus Creator1/8  "ax"
  Demux2/2 -> Bus Creator1/9  "zy"
  Demux2/3 -> Bus Creator1/10  "az"
  Bus Selector1/5 -> Bus Creator1/11  "<yaw>"
  Bus Selector1/6 -> Bus Creator1/12  "<yawspeed>"
  Bus Selector3/1 -> Bus Creator2/1  "<timestamp>"
  Bus Selector3/2 -> Gain1/1  "<roll>"
  Bus Selector3/3 -> Gain2/1  "<pitch>"
  Bus Selector3/4 -> Gain3/1  "<yaw>"
  Bus Selector3/5 -> Bus Creator2/5  "<thrust_body>"
  Gain1/1 -> Bus Creator2/2  "rollRate"
  Gain2/1 -> Bus Creator2/3  "pitchRate"
  Gain3/1 -> Bus Creator2/4  "yawRate"
  Bus Selector2/1 -> Bus Creator/4  "vehicle_attitude_setpoint"

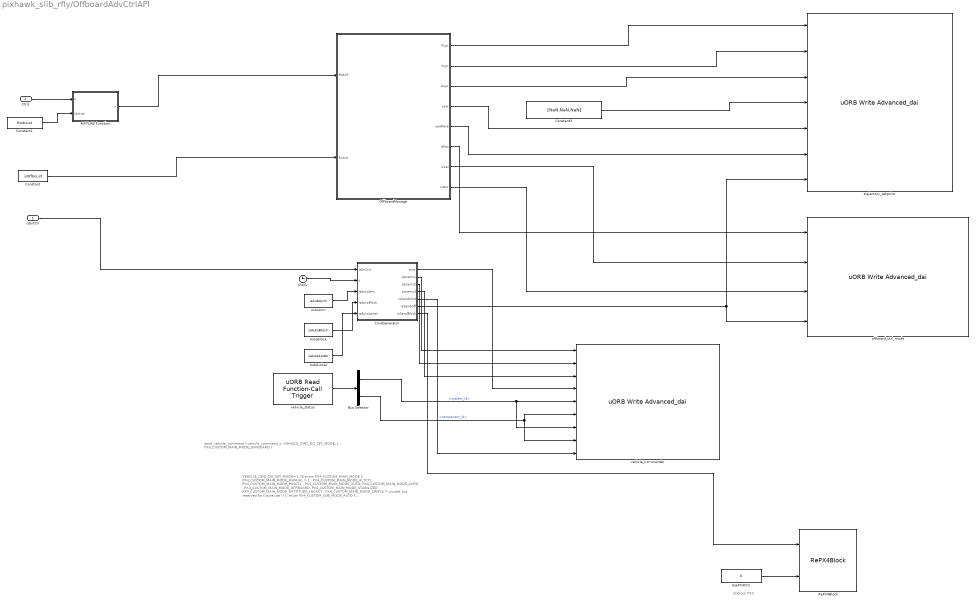
== system pixhawk_slib_rfly/OffboardAdvCtrlAPI ==
  note: VEHICLE_CMD_DO_SET_MODE= 1 76
      |
      | enum PX4_CUSTOM_MAIN_MODE {
      | PX4_CUSTOM_MAIN_MODE_MANUAL = 1 ,
      | PX4_CUSTOM_MAIN_MODE_ALTCTL ,
      | PX4_CUSTOM_MAIN_MODE_POSCTL ,
      | PX4_CUSTOM_MAIN_MODE_AUTO,
      | PX4_CUSTOM_MAIN_MODE_ACRO ,
      | PX4_CUSTOM_MAIN_MODE_OFFBOARD,
      | PX4_CUSTOM_MAIN_MODE_STABILIZED ,
      | PX4_CUSTOM_MAIN_MODE_RATTITUDE_LEGACY ,
      | PX4_CUSTOM_MAIN_MODE_SIMPLE /* unused, but reserved for future use */
      | };
      |
      | enum PX4_CUSTOM_SUB_MODE_AUTO {
      | PX4_CUSTOM_SUB_MODE_AUTO_READY = 1 ,
      | PX4_CUSTOM_SUB_MODE_AUTO_TAKEOFF ,
      | PX4_CUSTOM_SUB_MODE_AUTO_LOITER,
      | PX4_CUSTOM_SUB_MODE_AUTO_MISSION ,
      | PX4_CUSTOM_SUB_MODE_AUTO_RTL ,
      | PX4_CUSTOM_SUB_MODE_AUTO_LAND ,
      | PX4_CUSTOM_SUB_MODE_AUTO_RESERVED_DO_NOT_USE , // was PX4_CUSTOM_SUB_MODE_AUTO_RTGS, deleted 2020-03-05
      | PX4_CUSTOM_SUB_MODE_AUTO_FOLLOW_TARGET ,
      | PX4_CUSTOM_SUB_MODE_AUTO_PRECLAND
      | };
  note: Unblock PX4
  note: send_vehicle_command ( vehicle_command_s ::VEHICLE_CMD_DO_SET_MODE, 1 , PX4_CUSTOM_MAIN_MODE_OFFBOARD )
  isEnCtrl : Inport  OutDataTypeStr=boolean  PortDimensions=1
  Ctrls : Inport  Port=2  OutDataTypeStr=single  PortDimensions=4
  AutoArm : Constant  Value=isAutoArm  OutDataTypeStr=boolean
  AutoBlock : Constant  Value=isAutoBlock  OutDataTypeStr=boolean
  AutoLoiter : Constant  Value=isAutoLoiter  OutDataTypeStr=boolean
  Bus Selector : BusSelector  OutputSignals=system_id,component_id
  Clock : Clock
  CmdGenerator : MATLAB Function  TreatAsAtomicUnit=on  SystemSampleTime=SamTime
  Constant : Constant  Value=isOffEnList  OutDataTypeStr=boolean
  Constant1 : Constant  Value=EnIdxList
  Constant3 : Constant  Value=[NaN,NaN,NaN]  OutDataTypeStr=single
  MATLAB Function : MATLAB Function  TreatAsAtomicUnit=on  SystemSampleTime=SamTime
  OffboardManage : MATLAB Function  TreatAsAtomicUnit=on  SystemSampleTime=SamTime
  RePX4Block : $bdroot/RePX4Block  SamTime=SamTime
  UsePX4Ctrl : Constant  Value=0  OutDataTypeStr=uint8
  offboard_ctrl_mode : pixhawk_slib_uORB_RW/uORB Write Advanced_dai  Ts=0  uORB_AdvtQueue=on  uORB_FieldEnabledArr="0  0  0  1  0  0  0  0  0  0  0"  uORB_Topic_str=0  uORB_Topic_str_ID=0  uORB_Struct_DT="[1  1  1  1  1]"  BlockInputCount=5  uORB_StructParams="[\"voltage_v\",\"voltage_filtered_v\",\"current_a\",\"current_filtered_a\",\"remaining\"]"  uORB_PortSizes="[1  1  1  1]"  MsgSizeOf=0  MW_update=true
      settings: SourceProductName=Pixhawk Target Blocks
  trajectory_setpoint : pixhawk_slib_uORB_RW/uORB Write Advanced_dai  Ts=0  uORB_AdvtQueue=on  uORB_FieldEnabledArr="0  0  0  1  0  0  0  0  0  0  0"  uORB_Topic_str=0  uORB_Topic_str_ID=0  uORB_Struct_DT="[1  1  1  1  1]"  BlockInputCount=5  uORB_StructParams="[\"voltage_v\",\"voltage_filtered_v\",\"current_a\",\"current_filtered_a\",\"remaining\"]"  uORB_PortSizes="[1  1  1  1]"  MsgSizeOf=0  MW_update=true
      settings: SourceProductName=Pixhawk Target Blocks
  vehicle_commander : pixhawk_slib_uORB_RW/uORB Write Advanced_dai  Ts=0  uORB_AdvtQueue=on  uORB_FieldEnabledArr="0  0  0  1  0  0  0  0  0  0  0"  uORB_Topic_str=0  uORB_Topic_str_ID=0  uORB_Struct_DT="[1  1  1  1  1]"  BlockInputCount=5  uORB_StructParams="[\"voltage_v\",\"voltage_filtered_v\",\"current_a\",\"current_filtered_a\",\"remaining\"]"  uORB_PortSizes="[1  1  1  1]"  MsgSizeOf=0  MW_update=true
      settings: SourceProductName=Pixhawk Target Blocks
  vehicle_status : pixhawk_slib_uORB_RW/uORB Read Function-Call Trigger  uORB_Topic_str='vehicle_status'  BusObjVar=Bus: vehicle_status_SL  uORB_Interval=50  AsyncOutput=off  Fcn_call_select=Generate Function Call Signal  TaskName='Task1'  Poll_timeout=-1  Ts=SamTime
      settings: SourceProductName=Pixhawk Target Blocks
  wires:
  Ctrls/1 -> MATLAB Function/1(u)
  Constant1/1 -> MATLAB Function/2(idxList)
  Bus Selector/2 -> vehicle_commander/8, vehicle_commander/6  "<component_id>"
  CmdGenerator/5(isSendCmd) -> vehicle_commander/9
  Clock/1 -> CmdGenerator/2(t)
  Constant3/1 -> trajectory_setpoint/4
  OffboardManage/3(Axyz) -> trajectory_setpoint/3
  OffboardManage/6(isPos) -> offboard_ctrl_mode/1
  OffboardManage/7(isVel) -> offboard_ctrl_mode/2
  CmdGenerator/6(isSendOff) -> offboard_ctrl_mode/4, trajectory_setpoint/7
  AutoLoiter/1 -> CmdGenerator/5(isAutoLoiter)
  UsePX4Ctrl/1 -> RePX4Block/2
  AutoBlock/1 -> CmdGenerator/4(isAutoBlock)
  Constant/1 -> OffboardManage/2(EnList)
  CmdGenerator/4(params3) -> vehicle_commander/3
  CmdGenerator/1(cmd) -> vehicle_commander/4
  CmdGenerator/3(params2) -> vehicle_commander/2
  AutoArm/1 -> CmdGenerator/3(isAutoArm)
  OffboardManage/8(isAcc) -> offboard_ctrl_mode/3
  CmdGenerator/2(params1) -> vehicle_commander/1
  CmdGenerator/7(isSendBlock) -> RePX4Block/1
  OffboardManage/5(yawRate) -> trajectory_setpoint/6
  vehicle_status/1 -> Bus Selector/1
  OffboardManage/2(Vxyz) -> trajectory_setpoint/2
  OffboardManage/4(yaw) -> trajectory_setpoint/5
  OffboardManage/1(Pxyz) -> trajectory_setpoint/1
  MATLAB Function/1(y) -> OffboardManage/1(PVAYR)
  Bus Selector/1 -> vehicle_commander/7, vehicle_commander/5  "<system_id>"
  isEnCtrl/1 -> CmdGenerator/1(isEnCtrl)
